simulink model "schema_controllo_attritoStatico_CompDist"  (Simulink 8.8)
settings: Solver=VariableStepAuto  StartTime=0.0  StopTime=Tf  FixedStep=T  MaxStep=T  RelTol=1e-3  EnableMultiTasking=on
values from neighbouring files (symbols this model uses):
  Kr = diag(kr)    [calcolaDisturbo.m]
undefined symbols (not defined in the file or in its folder): bmStim, calcolaDisturboStim, dqData, Ka, km, Kp, kt, kta, ktp, ktv, Kv, kv, qData, Ra, T, Ta
CloseFcn:
  | rtwprivate ssgencode ModelCloseRequest ContributiCoppieComau
settings Model: Creator=Alessandro  LastModifiedBy=joecr  ExtModeAutoUpdateStatusClock=off
settings DataIOCC: OutputOption=SpecifiedOutputTimes  OutputTimes=[Ti:T:Tf]
settings OptimizationCC: ExpressionDepthLimit=2147483647  InitFltsAndDblsToZero=on
settings DebuggingCC: AlgebraicLoopMsg=none  SaveWithParameterizedLinksMsg=none  SignalResolutionControl=TryResolveAllWithWarning  SolverPrmCheckMsg=warning  InheritedTsInSrcMsg=none  MultiTaskDSMMsg=warning  MultiTaskCondExecSysMsg=none  TasksWithSamePriorityMsg=none  AllowSymbolicDim=off
settings GRTTargetCC: TargetFcnLib=ansi_tfl_tmw.mat

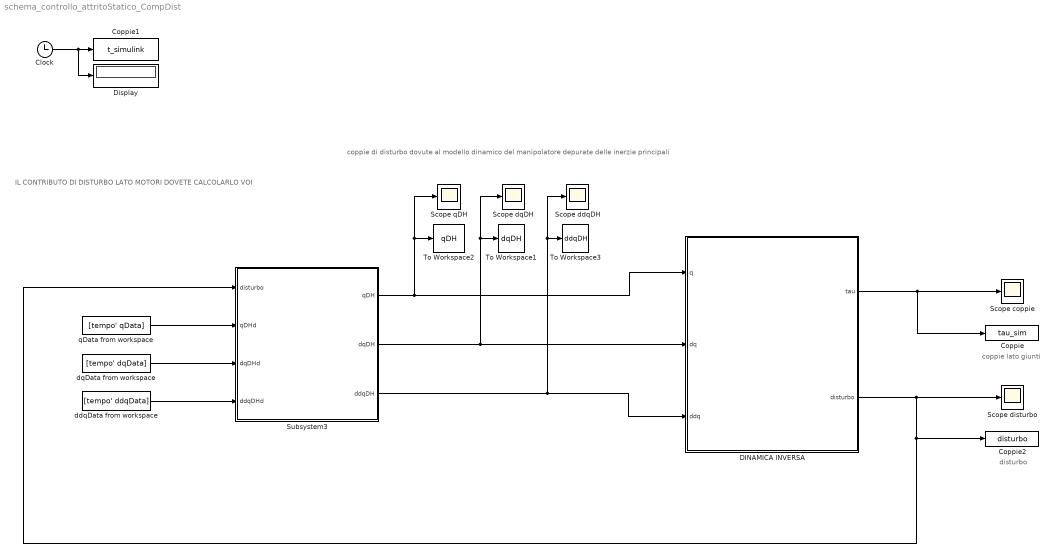
== system schema_controllo_attritoStatico_CompDist ==
  note: coppie di disturbo dovute al modello dinamico del manipolatore depurate delle inerzie principali
  note: coppie lato giunti
  note: IL CONTRIBUTO DI DISTURBO LATO MOTORI DOVETE CALCOLARLO VOI
  note: disturbo
  Clock : Clock
  Coppie : ToWorkspace  VariableName=tau_sim  SampleTime=-1
  Coppie1 : ToWorkspace  VariableName=t_simulink  SampleTime=-1
  Coppie2 : ToWorkspace  VariableName=disturbo  SampleTime=-1
  DINAMICA INVERSA : Subsystem
      mask Display:
      | disp('Contributi Coppie');
      | port_label('input', 1, 'qDH');
      | port_label('input', 2, 'dqDH');
      | port_label('input', 3, 'ddqDH');
      | port_label('output', 1, 'Coppie Complessive');
      | port_label('output', 2, 'Disturbo lato motori');
  Display : Display
  Scope coppie : Scope
  Scope ddqDH : Scope
  Scope disturbo : Scope
  Scope dqDH : Scope
  Scope qDH : Scope
  Subsystem3 : Subsystem
      mask Display:
      | disp('Controllo');
      | port_label('input', 1, 'disturbo');
      | port_label('input', 2, 'qDHd');
      | port_label('input', 3, 'dqDHd');
      | port_label('input', 4, 'ddqDHd');
      | port_label('output', 1, 'qDH');
      | port_label('output', 2, 'dqDH');
      | port_label('output', 3, 'ddqDH');
  To Workspace1 : ToWorkspace  VariableName=dqDH  SampleTime=-1
  To Workspace2 : ToWorkspace  VariableName=qDH  SampleTime=-1
  To Workspace3 : ToWorkspace  VariableName=ddqDH  SampleTime=-1
  ddqData from workspace : FromWorkspace  VariableName=[tempo' ddqData]  OutputAfterFinalValue=Holding final value
  dqData from workspace : FromWorkspace  VariableName=[tempo' dqData]  OutputAfterFinalValue=Holding final value
  qData from workspace : FromWorkspace  VariableName=[tempo' qData]  OutputAfterFinalValue=Holding final value
  wires:
  Clock/1 -> Coppie1/1, Display/1
  Subsystem3/2(dqDH) -> To Workspace1/1, Scope dqDH/1, DINAMICA INVERSA/2(dq)
  DINAMICA INVERSA/1(tau) -> Coppie/1, Scope coppie/1
  Subsystem3/1(qDH) -> DINAMICA INVERSA/1(q), To Workspace2/1, Scope qDH/1
  Subsystem3/3(ddqDH) -> DINAMICA INVERSA/3(ddq), To Workspace3/1, Scope ddqDH/1
  DINAMICA INVERSA/2(disturbo) -> Subsystem3/1(disturbo), Coppie2/1, Scope disturbo/1
  qData from workspace/1 -> Subsystem3/2(qDHd)
  dqData from workspace/1 -> Subsystem3/3(dqDHd)
  ddqData from workspace/1 -> Subsystem3/4(ddqDHd)

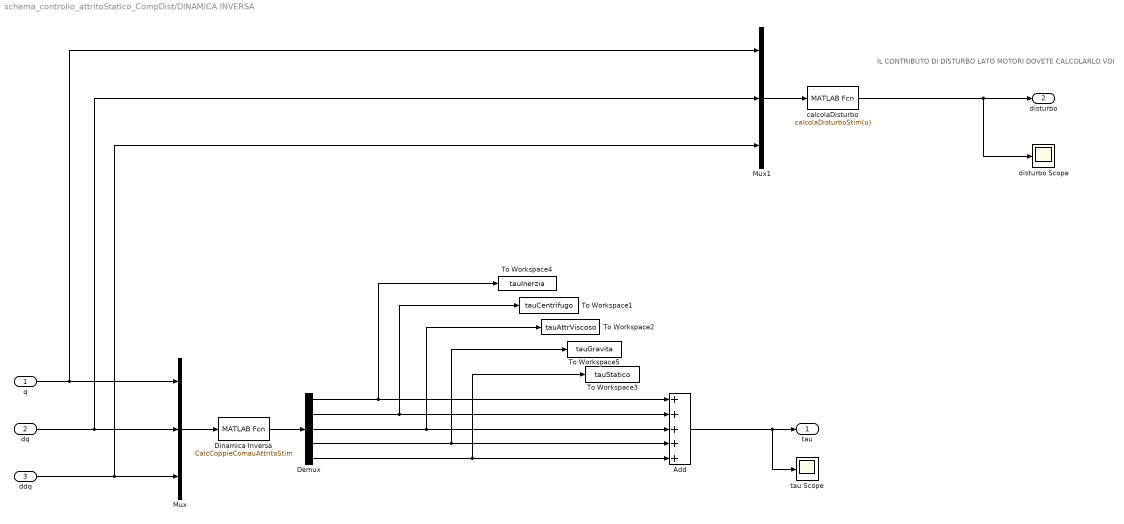
== system schema_controllo_attritoStatico_CompDist/DINAMICA INVERSA ==
  note: IL CONTRIBUTO DI DISTURBO LATO MOTORI DOVETE CALCOLARLO VOI
  q : Inport
  dq : Inport  Port=2
  ddq : Inport  Port=3
  Add : Sum  Inputs=+++++
  Demux : Demux  Outputs=5
  Dinamica Inversa : MATLABFcn  MATLABFcn=CalcCoppieComauAttritoStim  OutputDimensions=30
  Mux : Mux  Inputs=3
  Mux1 : Mux  Inputs=3
  To Workspace1 : ToWorkspace  VariableName=tauCentrifugo  SampleTime=-1
  To Workspace2 : ToWorkspace  VariableName=tauAttrViscoso  SampleTime=-1
  To Workspace3 : ToWorkspace  VariableName=tauStatico  SampleTime=-1
  To Workspace4 : ToWorkspace  VariableName=tauInerzia  SampleTime=-1
  To Workspace5 : ToWorkspace  VariableName=tauGravita  SampleTime=-1
  calcolaDisturbo : MATLABFcn  MATLABFcn=calcolaDisturboStim(u)  OutputDimensions=6
  disturbo Scope : Scope
  tau Scope : Scope
  tau : Outport
  disturbo : Outport  Port=2
  wires:
  Mux/1 -> Dinamica Inversa/1
  ddq/1 -> Mux1/3, Mux/3
  Dinamica Inversa/1 -> Demux/1
  Demux/1 -> To Workspace4/1, Add/1
  Demux/3 -> Add/3, To Workspace2/1
  Demux/4 -> Add/4, To Workspace5/1
  calcolaDisturbo/1 -> disturbo Scope/1, disturbo/1
  Mux1/1 -> calcolaDisturbo/1
  Demux/2 -> Add/2, To Workspace1/1
  Add/1 -> tau Scope/1, tau/1
  q/1 -> Mux1/1, Mux/1
  dq/1 -> Mux1/2, Mux/2
  Demux/5 -> To Workspace3/1, Add/5

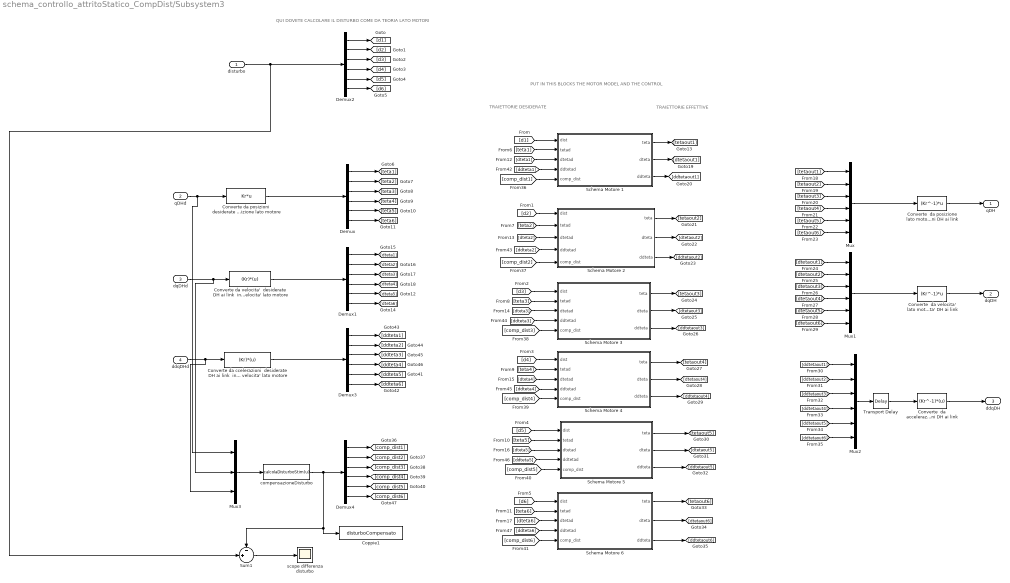
== system schema_controllo_attritoStatico_CompDist/Subsystem3 ==
  note: PUT IN THIS BLOCKS THE MOTOR MODEL AND THE CONTROL
  note: TRAIETTORIE DESIDERATE
  note: TRAIETTORIE EFFETTIVE
  note: QUI DOVETE CALCOLARE IL DISTURBO COME DA TEORIA LATO MOTORI
  disturbo : Inport
  qDHd : Inport  Port=2
  dqDHd : Inport  Port=3
  ddqDHd : Inport  Port=4
  Converte  da accelerazioni lato motore  ad accelerazioni DH ai link : MATLABFcn  MATLABFcn=(Kr^-1)*(u)
  "Converte  da posizione lato motore a  posizioni DH ai link " : MATLABFcn  MATLABFcn=(Kr^-1)*u
  "Converte  da velocita' lato motore  a velocita' DH ai link " : MATLABFcn  MATLABFcn=(Kr^-1)*u
  Converte da ccelerazioni  desiderate DH ai link  in velocita' lato motore : MATLABFcn  MATLABFcn=(Kr)*(u)
  "Converte da posizioni  desiderate DH ai link  in posizione lato motore " : MATLABFcn  MATLABFcn=Kr*u
  "Converte da velocita'  desiderate DH ai link  in velocita' lato motore " : MATLABFcn  MATLABFcn=(Kr)*(u)
  Coppie1 : ToWorkspace  VariableName=disturboCompensato  SampleTime=-1
  Demux{,1..4} (5 alike) : Demux  Outputs=6
  Mux : Mux  Inputs=6
  Mux1 : Mux  Inputs=6
  Mux2 : Mux  Inputs=6
  Mux3 : Mux  Inputs=3
  Schema Motore 1 : Subsystem  mask{i=1}
  Schema Motore 2 : Subsystem  mask{i=2}
  Schema Motore 3 : Subsystem  mask{i=3}
  Schema Motore 4 : Subsystem  mask{i=4}
  Schema Motore 5 : Subsystem  mask{i=5}
  Schema Motore 6 : Subsystem  mask{i=6}
  Sum1 : Sum  Inputs=-+|
  Transport Delay : TransportDelay  DelayTime=T
  compensazioneDisturbo : MATLABFcn  MATLABFcn=calcolaDisturboStim(u)
  scope differenza disturbo : Scope
  qDH : Outport
  dqDH : Outport  Port=2
  ddqDH : Outport  Port=3
  wires:
  qDHd/1 -> Mux3/1, "Converte da posizioni  desiderate DH ai link  in posizione lato motore "/1
  dqDHd/1 -> Mux3/2, "Converte da velocita'  desiderate DH ai link  in velocita' lato motore "/1
  "Converte  da velocita' lato motore  a velocita' DH ai link "/1 -> dqDH/1
  Converte  da accelerazioni lato motore  ad accelerazioni DH ai link/1 -> ddqDH/1
  "Converte da posizioni  desiderate DH ai link  in posizione lato motore "/1 -> Demux/1
  disturbo/1 -> Sum1/2, Demux2/1
  "Converte  da posizione lato motore a  posizioni DH ai link "/1 -> qDH/1
  Mux/1 -> "Converte  da posizione lato motore a  posizioni DH ai link "/1
  Demux2/1 -> [d1]
  Demux2/2 -> [d2]
  Demux2/3 -> [d3]
  Demux2/4 -> [d4]
  Demux2/5 -> [d5]
  Demux2/6 -> [d6]
  [d3] -> Schema Motore 3/1(dist)
  [d4] -> Schema Motore 4/1(dist)
  [d5] -> Schema Motore 5/1(dist)
  [d6] -> Schema Motore 6/1(dist)
  Demux/1 -> [teta1]
  Demux/2 -> [teta2]
  Demux/3 -> [teta3]
  Demux/4 -> [teta4]
  Demux/5 -> [teta5]
  Demux/6 -> [teta6]
  [teta2] -> Schema Motore 2/2(tetad)
  [teta3] -> Schema Motore 3/2(tetad)
  [teta4] -> Schema Motore 4/2(tetad)
  [teta5] -> Schema Motore 5/2(tetad)
  [teta6] -> Schema Motore 6/2(tetad)
  "Converte da velocita'  desiderate DH ai link  in velocita' lato motore "/1 -> Demux1/1
  Demux1/1 -> [dteta1]
  Demux1/2 -> [dteta2]
  Demux1/3 -> [dteta3]
  Demux1/4 -> [dteta4]
  Demux1/5 -> [dteta5]
  Demux1/6 -> [dteta6]
  [dteta2] -> Schema Motore 2/3(dtetad)
  [tetaout1] -> Mux/1
  [tetaout2] -> Mux/2
  [tetaout3] -> Mux/3
  [tetaout4] -> Mux/4
  [tetaout5] -> Mux/5
  [tetaout6] -> Mux/6
  Mux1/1 -> "Converte  da velocita' lato motore  a velocita' DH ai link "/1
  [dtetaout1] -> Mux1/1
  [dtetaout2] -> Mux1/2
  [dtetaout3] -> Mux1/3
  [dtetaout4] -> Mux1/4
  [dtetaout5] -> Mux1/5
  [dtetaout6] -> Mux1/6
  Mux2/1 -> Transport Delay/1
  [ddtetaout1] -> Mux2/1
  [ddtetaout2] -> Mux2/2
  [ddtetaout3] -> Mux2/3
  [ddtetaout4] -> Mux2/4
  [ddtetaout5] -> Mux2/5
  [ddtetaout6] -> Mux2/6
  Schema Motore 2/1(teta) -> [tetaout2]
  Schema Motore 2/2(dteta) -> [dtetaout2]
  Transport Delay/1 -> Converte  da accelerazioni lato motore  ad accelerazioni DH ai link/1
  [teta1] -> Schema Motore 1/2(tetad)
  [dteta1] -> Schema Motore 1/3(dtetad)
  Schema Motore 1/1(teta) -> [tetaout1]
  Schema Motore 1/2(dteta) -> [dtetaout1]
  Schema Motore 1/3(ddteta) -> [ddtetaout1]
  [d1] -> Schema Motore 1/1(dist)
  ddqDHd/1 -> Mux3/3, Converte da ccelerazioni  desiderate DH ai link  in velocita' lato motore/1
  Demux3/1 -> [ddteta1]
  Demux3/2 -> [ddteta2]
  Demux3/3 -> [ddteta3]
  Demux3/4 -> [ddteta4]
  Demux3/5 -> [ddteta5]
  Demux3/6 -> [ddteta6]
  Converte da ccelerazioni  desiderate DH ai link  in velocita' lato motore/1 -> Demux3/1
  [ddteta1] -> Schema Motore 1/4(ddtetad)
  Schema Motore 3/1(teta) -> [tetaout3]
  Schema Motore 3/2(dteta) -> [dtetaout3]
  Schema Motore 3/3(ddteta) -> [ddtetaout3]
  Schema Motore 4/1(teta) -> [tetaout4]
  Schema Motore 4/2(dteta) -> [dtetaout4]
  Schema Motore 4/3(ddteta) -> [ddtetaout4]
  Schema Motore 5/1(teta) -> [tetaout5]
  Schema Motore 5/2(dteta) -> [dtetaout5]
  Schema Motore 5/3(ddteta) -> [ddtetaout5]
  Schema Motore 6/1(teta) -> [tetaout6]
  Schema Motore 6/2(dteta) -> [dtetaout6]
  Schema Motore 6/3(ddteta) -> [ddtetaout6]
  [ddteta2] -> Schema Motore 2/4(ddtetad)
  [dteta4] -> Schema Motore 4/3(dtetad)
  [ddteta4] -> Schema Motore 4/4(ddtetad)
  [ddteta3] -> Schema Motore 3/4(ddtetad)
  [dteta3] -> Schema Motore 3/3(dtetad)
  [d2] -> Schema Motore 2/1(dist)
  Schema Motore 2/3(ddteta) -> [ddtetaout2]
  [dteta5] -> Schema Motore 5/3(dtetad)
  [ddteta5] -> Schema Motore 5/4(ddtetad)
  [dteta6] -> Schema Motore 6/3(dtetad)
  [ddteta6] -> Schema Motore 6/4(ddtetad)
  [comp_dist1] -> Schema Motore 1/5(comp_dist)
  Demux4/1 -> [comp_dist1]
  Demux4/2 -> [comp_dist2]
  Demux4/3 -> [comp_dist3]
  Demux4/4 -> [comp_dist4]
  Demux4/5 -> [comp_dist5]
  Demux4/6 -> [comp_dist6]
  Mux3/1 -> compensazioneDisturbo/1
  [comp_dist2] -> Schema Motore 2/5(comp_dist)
  [comp_dist6] -> Schema Motore 6/5(comp_dist)
  [comp_dist5] -> Schema Motore 5/5(comp_dist)
  [comp_dist4] -> Schema Motore 4/5(comp_dist)
  [comp_dist3] -> Schema Motore 3/5(comp_dist)
  compensazioneDisturbo/1 -> Sum1/1, Coppie1/1, Demux4/1
  Sum1/1 -> scope differenza disturbo/1

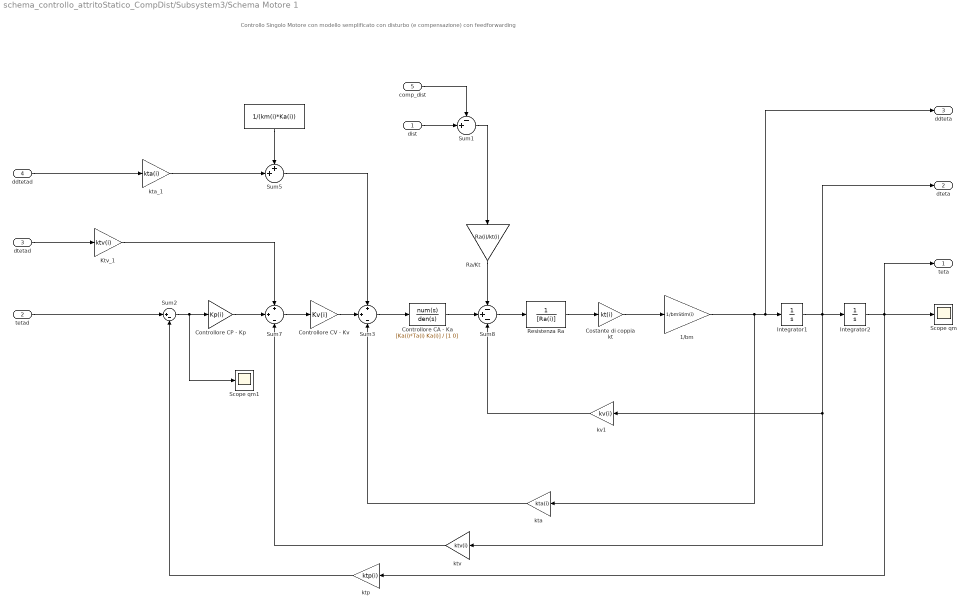
== system schema_controllo_attritoStatico_CompDist/Subsystem3/Schema Motore 1 ==
  note: Controllo Singolo Motore con modello semplificato con disturbo (e compensazione) con feedforwarding
  dist : Inport  PortDimensions=1
  tetad : Inport  Port=2  PortDimensions=1
  dtetad : Inport  Port=3  PortDimensions=1
  ddtetad : Inport  Port=4  PortDimensions=1
  comp_dist : Inport  Port=5  PortDimensions=1
  " " : Constant  Value=1/(km(i)*Ka(i))
  " Controllore CV - Kv" : Gain  Gain=Kv(i)
  1/bm : Gain  Gain=1/bmStim(i)
  Controllore CA - Ka : TransferFcn  Numerator=[Ka(i)*Ta(i) Ka(i)]  Denominator=[1 0]
  Controllore CP - Kp : Gain  Gain=Kp(i)
  Costante di coppia kt : Gain  Gain=kt(i)
  Integrator1 : Integrator  InitialCondition=Kr(i,i)*dqData(1,i)
  "Integrator2 " : Integrator  InitialCondition=Kr(i,i)*qData(1,i)
  Ktv_1 : Gain  Gain=ktv(i)
  Ra/Kt : Gain  Gain=Ra(i)/kt(i)
  "Resistenza Ra " : TransferFcn  Denominator=[Ra(i)]
  Scope qm : Scope
  Scope qm1 : Scope
  Sum1 : Sum  Inputs=-+|
  Sum2 : Sum  Inputs=|+-
  Sum3 : Sum  Inputs=+|+|-
  Sum5 : Sum  Inputs=++|
  Sum7 : Sum  Inputs=+|+|-
  Sum8 : Sum  Inputs=-+-
  kta : Gain  Gain=kta(i)
  kta_1 : Gain  Gain=kta(i)
  ktp : Gain  Gain=ktp(i)
  ktv : Gain  Gain=ktv(i)
  kv1 : Gain  Gain=kv(i)
  teta : Outport  PortDimensions=1
  dteta : Outport  Port=2  PortDimensions=1
  ddteta : Outport  Port=3  PortDimensions=1
  wires:
  Sum7/1 -> " Controllore CV - Kv"/1
  Sum3/1 -> Controllore CA - Ka/1
  ktp/1 -> Sum2/2
  tetad/1 -> Sum2/1
  Sum8/1 -> "Resistenza Ra "/1
  kv1/1 -> Sum8/3
  Integrator1/1 -> dteta/1, ktv/1, kv1/1, "Integrator2 "/1
  "Resistenza Ra "/1 -> Costante di coppia kt/1
  Costante di coppia kt/1 -> 1/bm/1
  Controllore CP - Kp/1 -> Sum7/2
  Ktv_1/1 -> Sum7/1
  ktv/1 -> Sum7/3
  " Controllore CV - Kv"/1 -> Sum3/2
  kta_1/1 -> Sum5/2
  " "/1 -> Sum5/1
  Sum5/1 -> Sum3/1
  ddtetad/1 -> kta_1/1
  dtetad/1 -> Ktv_1/1
  "Integrator2 "/1 -> ktp/1, teta/1, Scope qm/1
  kta/1 -> Sum3/3
  1/bm/1 -> kta/1, ddteta/1, Integrator1/1
  Ra/Kt/1 -> Sum8/1
  Controllore CA - Ka/1 -> Sum8/2
  comp_dist/1 -> Sum1/1
  Sum2/1 -> Scope qm1/1, Controllore CP - Kp/1
  dist/1 -> Sum1/2
  Sum1/1 -> Ra/Kt/1

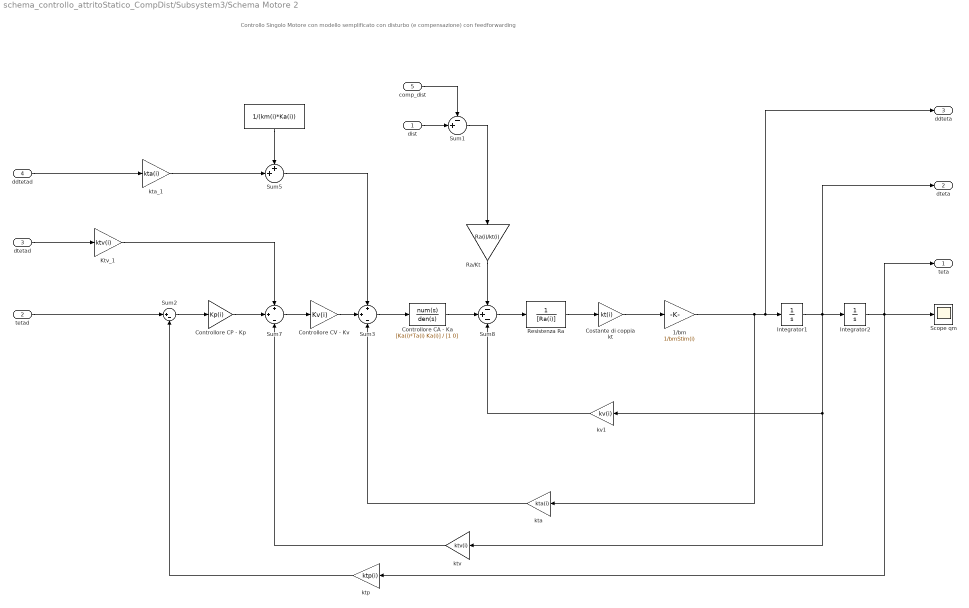
== system schema_controllo_attritoStatico_CompDist/Subsystem3/Schema Motore 2 ==
  note: Controllo Singolo Motore con modello semplificato con disturbo (e compensazione) con feedforwarding
  dist : Inport  PortDimensions=1
  tetad : Inport  Port=2  PortDimensions=1
  dtetad : Inport  Port=3  PortDimensions=1
  ddtetad : Inport  Port=4  PortDimensions=1
  comp_dist : Inport  Port=5  PortDimensions=1
  " " : Constant  Value=1/(km(i)*Ka(i))
  " Controllore CV - Kv" : Gain  Gain=Kv(i)
  1/bm : Gain  Gain=1/bmStim(i)
  Controllore CA - Ka : TransferFcn  Numerator=[Ka(i)*Ta(i) Ka(i)]  Denominator=[1 0]
  Controllore CP - Kp : Gain  Gain=Kp(i)
  Costante di coppia kt : Gain  Gain=kt(i)
  Integrator1 : Integrator  InitialCondition=Kr(i,i)*dqData(1,i)
  "Integrator2 " : Integrator  InitialCondition=Kr(i,i)*qData(1,i)
  Ktv_1 : Gain  Gain=ktv(i)
  Ra/Kt : Gain  Gain=Ra(i)/kt(i)
  "Resistenza Ra " : TransferFcn  Denominator=[Ra(i)]
  Scope qm : Scope
  Sum1 : Sum  Inputs=-+|
  Sum2 : Sum  Inputs=|+-
  Sum3 : Sum  Inputs=+|+|-
  Sum5 : Sum  Inputs=++|
  Sum7 : Sum  Inputs=+|+|-
  Sum8 : Sum  Inputs=-+-
  kta : Gain  Gain=kta(i)
  kta_1 : Gain  Gain=kta(i)
  ktp : Gain  Gain=ktp(i)
  ktv : Gain  Gain=ktv(i)
  kv1 : Gain  Gain=kv(i)
  teta : Outport  PortDimensions=1
  dteta : Outport  Port=2  PortDimensions=1
  ddteta : Outport  Port=3  PortDimensions=1
  wires:
  Sum7/1 -> " Controllore CV - Kv"/1
  Sum3/1 -> Controllore CA - Ka/1
  ktp/1 -> Sum2/2
  tetad/1 -> Sum2/1
  Sum8/1 -> "Resistenza Ra "/1
  kv1/1 -> Sum8/3
  Integrator1/1 -> dteta/1, ktv/1, kv1/1, "Integrator2 "/1
  "Resistenza Ra "/1 -> Costante di coppia kt/1
  Costante di coppia kt/1 -> 1/bm/1
  Controllore CP - Kp/1 -> Sum7/2
  Ktv_1/1 -> Sum7/1
  ktv/1 -> Sum7/3
  " Controllore CV - Kv"/1 -> Sum3/2
  kta_1/1 -> Sum5/2
  " "/1 -> Sum5/1
  Sum5/1 -> Sum3/1
  ddtetad/1 -> kta_1/1
  dtetad/1 -> Ktv_1/1
  "Integrator2 "/1 -> ktp/1, teta/1, Scope qm/1
  kta/1 -> Sum3/3
  Sum2/1 -> Controllore CP - Kp/1
  1/bm/1 -> ddteta/1, Integrator1/1, kta/1
  Ra/Kt/1 -> Sum8/1
  Controllore CA - Ka/1 -> Sum8/2
  dist/1 -> Sum1/2
  comp_dist/1 -> Sum1/1
  Sum1/1 -> Ra/Kt/1

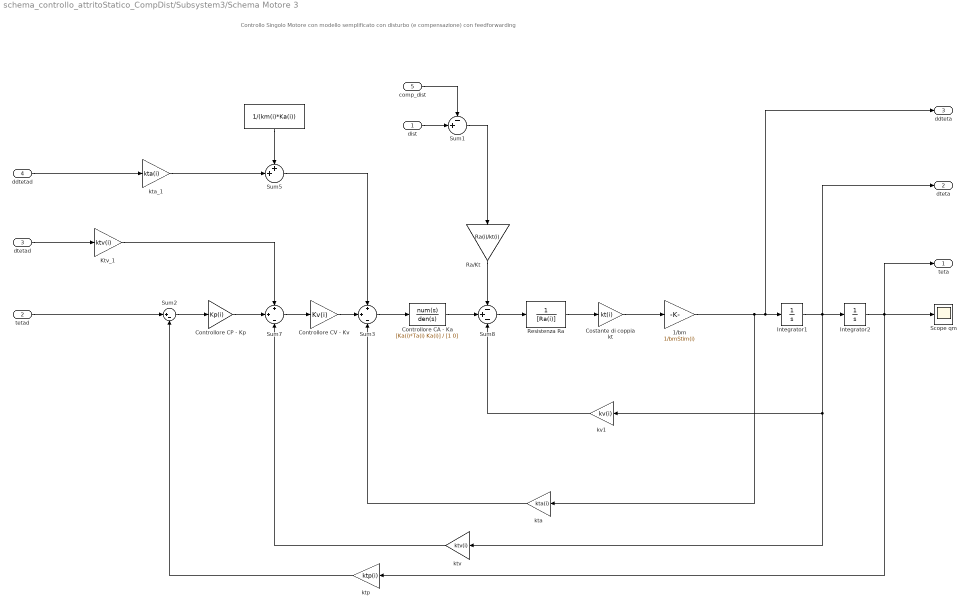
== system schema_controllo_attritoStatico_CompDist/Subsystem3/Schema Motore 3 ==
  note: Controllo Singolo Motore con modello semplificato con disturbo (e compensazione) con feedforwarding
  dist : Inport  PortDimensions=1
  tetad : Inport  Port=2  PortDimensions=1
  dtetad : Inport  Port=3  PortDimensions=1
  ddtetad : Inport  Port=4  PortDimensions=1
  comp_dist : Inport  Port=5  PortDimensions=1
  " " : Constant  Value=1/(km(i)*Ka(i))
  " Controllore CV - Kv" : Gain  Gain=Kv(i)
  1/bm : Gain  Gain=1/bmStim(i)
  Controllore CA - Ka : TransferFcn  Numerator=[Ka(i)*Ta(i) Ka(i)]  Denominator=[1 0]
  Controllore CP - Kp : Gain  Gain=Kp(i)
  Costante di coppia kt : Gain  Gain=kt(i)
  Integrator1 : Integrator  InitialCondition=Kr(i,i)*dqData(1,i)
  "Integrator2 " : Integrator  InitialCondition=Kr(i,i)*qData(1,i)
  Ktv_1 : Gain  Gain=ktv(i)
  Ra/Kt : Gain  Gain=Ra(i)/kt(i)
  "Resistenza Ra " : TransferFcn  Denominator=[Ra(i)]
  Scope qm : Scope
  Sum1 : Sum  Inputs=-+|
  Sum2 : Sum  Inputs=|+-
  Sum3 : Sum  Inputs=+|+|-
  Sum5 : Sum  Inputs=++|
  Sum7 : Sum  Inputs=+|+|-
  Sum8 : Sum  Inputs=-+-
  kta : Gain  Gain=kta(i)
  kta_1 : Gain  Gain=kta(i)
  ktp : Gain  Gain=ktp(i)
  ktv : Gain  Gain=ktv(i)
  kv1 : Gain  Gain=kv(i)
  teta : Outport  PortDimensions=1
  dteta : Outport  Port=2  PortDimensions=1
  ddteta : Outport  Port=3  PortDimensions=1
  wires:
  Sum7/1 -> " Controllore CV - Kv"/1
  Sum3/1 -> Controllore CA - Ka/1
  ktp/1 -> Sum2/2
  tetad/1 -> Sum2/1
  Sum8/1 -> "Resistenza Ra "/1
  kv1/1 -> Sum8/3
  Integrator1/1 -> dteta/1, ktv/1, kv1/1, "Integrator2 "/1
  "Resistenza Ra "/1 -> Costante di coppia kt/1
  Costante di coppia kt/1 -> 1/bm/1
  Controllore CP - Kp/1 -> Sum7/2
  Ktv_1/1 -> Sum7/1
  ktv/1 -> Sum7/3
  " Controllore CV - Kv"/1 -> Sum3/2
  kta_1/1 -> Sum5/2
  " "/1 -> Sum5/1
  Sum5/1 -> Sum3/1
  ddtetad/1 -> kta_1/1
  dtetad/1 -> Ktv_1/1
  "Integrator2 "/1 -> ktp/1, teta/1, Scope qm/1
  kta/1 -> Sum3/3
  Sum2/1 -> Controllore CP - Kp/1
  1/bm/1 -> ddteta/1, Integrator1/1, kta/1
  Ra/Kt/1 -> Sum8/1
  Controllore CA - Ka/1 -> Sum8/2
  dist/1 -> Sum1/2
  comp_dist/1 -> Sum1/1
  Sum1/1 -> Ra/Kt/1

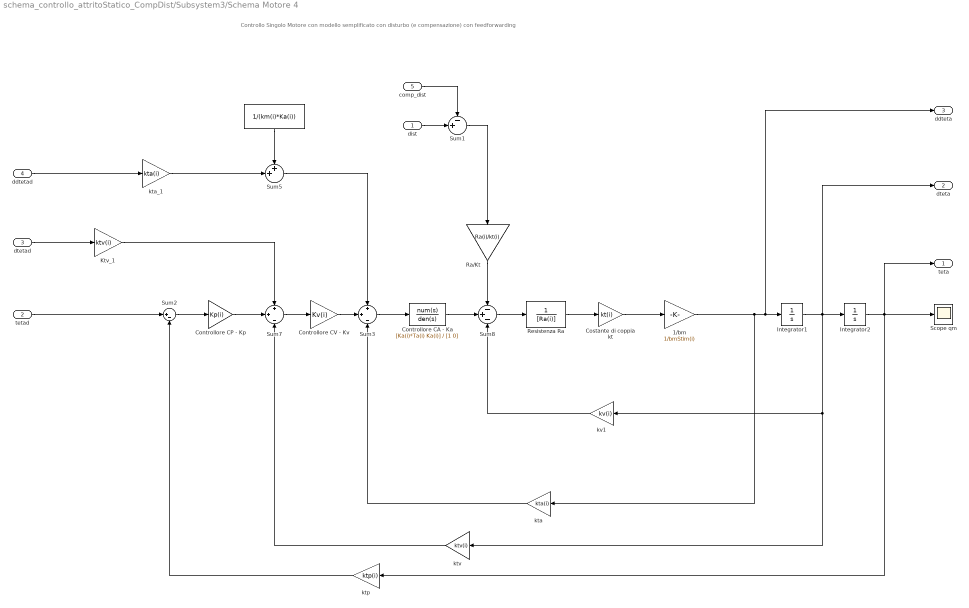
== system schema_controllo_attritoStatico_CompDist/Subsystem3/Schema Motore 4 ==
  note: Controllo Singolo Motore con modello semplificato con disturbo (e compensazione) con feedforwarding
  dist : Inport  PortDimensions=1
  tetad : Inport  Port=2  PortDimensions=1
  dtetad : Inport  Port=3  PortDimensions=1
  ddtetad : Inport  Port=4  PortDimensions=1
  comp_dist : Inport  Port=5  PortDimensions=1
  " " : Constant  Value=1/(km(i)*Ka(i))
  " Controllore CV - Kv" : Gain  Gain=Kv(i)
  1/bm : Gain  Gain=1/bmStim(i)
  Controllore CA - Ka : TransferFcn  Numerator=[Ka(i)*Ta(i) Ka(i)]  Denominator=[1 0]
  Controllore CP - Kp : Gain  Gain=Kp(i)
  Costante di coppia kt : Gain  Gain=kt(i)
  Integrator1 : Integrator  InitialCondition=Kr(i,i)*dqData(1,i)
  "Integrator2 " : Integrator  InitialCondition=Kr(i,i)*qData(1,i)
  Ktv_1 : Gain  Gain=ktv(i)
  Ra/Kt : Gain  Gain=Ra(i)/kt(i)
  "Resistenza Ra " : TransferFcn  Denominator=[Ra(i)]
  Scope qm : Scope
  Sum1 : Sum  Inputs=-+|
  Sum2 : Sum  Inputs=|+-
  Sum3 : Sum  Inputs=+|+|-
  Sum5 : Sum  Inputs=++|
  Sum7 : Sum  Inputs=+|+|-
  Sum8 : Sum  Inputs=-+-
  kta : Gain  Gain=kta(i)
  kta_1 : Gain  Gain=kta(i)
  ktp : Gain  Gain=ktp(i)
  ktv : Gain  Gain=ktv(i)
  kv1 : Gain  Gain=kv(i)
  teta : Outport  PortDimensions=1
  dteta : Outport  Port=2  PortDimensions=1
  ddteta : Outport  Port=3  PortDimensions=1
  wires:
  Sum7/1 -> " Controllore CV - Kv"/1
  Sum3/1 -> Controllore CA - Ka/1
  ktp/1 -> Sum2/2
  tetad/1 -> Sum2/1
  Sum8/1 -> "Resistenza Ra "/1
  kv1/1 -> Sum8/3
  Integrator1/1 -> dteta/1, ktv/1, kv1/1, "Integrator2 "/1
  "Resistenza Ra "/1 -> Costante di coppia kt/1
  Costante di coppia kt/1 -> 1/bm/1
  Controllore CP - Kp/1 -> Sum7/2
  Ktv_1/1 -> Sum7/1
  ktv/1 -> Sum7/3
  " Controllore CV - Kv"/1 -> Sum3/2
  kta_1/1 -> Sum5/2
  " "/1 -> Sum5/1
  Sum5/1 -> Sum3/1
  ddtetad/1 -> kta_1/1
  dtetad/1 -> Ktv_1/1
  "Integrator2 "/1 -> ktp/1, teta/1, Scope qm/1
  kta/1 -> Sum3/3
  Sum2/1 -> Controllore CP - Kp/1
  1/bm/1 -> ddteta/1, Integrator1/1, kta/1
  Ra/Kt/1 -> Sum8/1
  Controllore CA - Ka/1 -> Sum8/2
  dist/1 -> Sum1/2
  comp_dist/1 -> Sum1/1
  Sum1/1 -> Ra/Kt/1

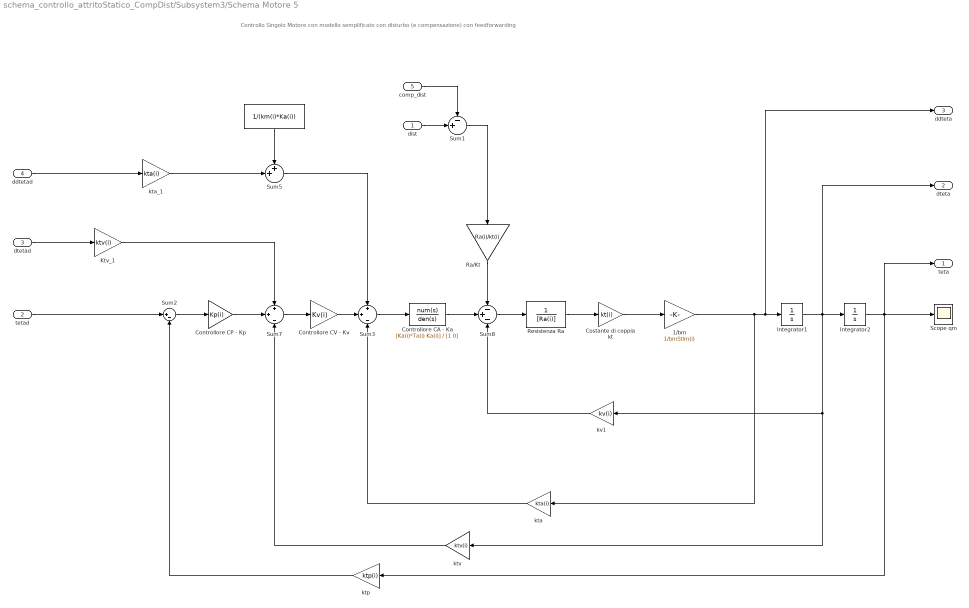
== system schema_controllo_attritoStatico_CompDist/Subsystem3/Schema Motore 5 ==
  note: Controllo Singolo Motore con modello semplificato con disturbo (e compensazione) con feedforwarding
  dist : Inport  PortDimensions=1
  tetad : Inport  Port=2  PortDimensions=1
  dtetad : Inport  Port=3  PortDimensions=1
  ddtetad : Inport  Port=4  PortDimensions=1
  comp_dist : Inport  Port=5  PortDimensions=1
  " " : Constant  Value=1/(km(i)*Ka(i))
  " Controllore CV - Kv" : Gain  Gain=Kv(i)
  1/bm : Gain  Gain=1/bmStim(i)
  Controllore CA - Ka : TransferFcn  Numerator=[Ka(i)*Ta(i) Ka(i)]  Denominator=[1 0]
  Controllore CP - Kp : Gain  Gain=Kp(i)
  Costante di coppia kt : Gain  Gain=kt(i)
  Integrator1 : Integrator  InitialCondition=Kr(i,i)*dqData(1,i)
  "Integrator2 " : Integrator  InitialCondition=Kr(i,i)*qData(1,i)
  Ktv_1 : Gain  Gain=ktv(i)
  Ra/Kt : Gain  Gain=Ra(i)/kt(i)
  "Resistenza Ra " : TransferFcn  Denominator=[Ra(i)]
  Scope qm : Scope
  Sum1 : Sum  Inputs=-+|
  Sum2 : Sum  Inputs=|+-
  Sum3 : Sum  Inputs=+|+|-
  Sum5 : Sum  Inputs=++|
  Sum7 : Sum  Inputs=+|+|-
  Sum8 : Sum  Inputs=-+-
  kta : Gain  Gain=kta(i)
  kta_1 : Gain  Gain=kta(i)
  ktp : Gain  Gain=ktp(i)
  ktv : Gain  Gain=ktv(i)
  kv1 : Gain  Gain=kv(i)
  teta : Outport  PortDimensions=1
  dteta : Outport  Port=2  PortDimensions=1
  ddteta : Outport  Port=3  PortDimensions=1
  wires:
  Sum7/1 -> " Controllore CV - Kv"/1
  Sum3/1 -> Controllore CA - Ka/1
  ktp/1 -> Sum2/2
  tetad/1 -> Sum2/1
  Sum8/1 -> "Resistenza Ra "/1
  kv1/1 -> Sum8/3
  Integrator1/1 -> dteta/1, ktv/1, kv1/1, "Integrator2 "/1
  "Resistenza Ra "/1 -> Costante di coppia kt/1
  Costante di coppia kt/1 -> 1/bm/1
  Controllore CP - Kp/1 -> Sum7/2
  Ktv_1/1 -> Sum7/1
  ktv/1 -> Sum7/3
  " Controllore CV - Kv"/1 -> Sum3/2
  kta_1/1 -> Sum5/2
  " "/1 -> Sum5/1
  Sum5/1 -> Sum3/1
  ddtetad/1 -> kta_1/1
  dtetad/1 -> Ktv_1/1
  "Integrator2 "/1 -> ktp/1, teta/1, Scope qm/1
  kta/1 -> Sum3/3
  Sum2/1 -> Controllore CP - Kp/1
  1/bm/1 -> ddteta/1, Integrator1/1, kta/1
  Ra/Kt/1 -> Sum8/1
  Controllore CA - Ka/1 -> Sum8/2
  dist/1 -> Sum1/2
  comp_dist/1 -> Sum1/1
  Sum1/1 -> Ra/Kt/1

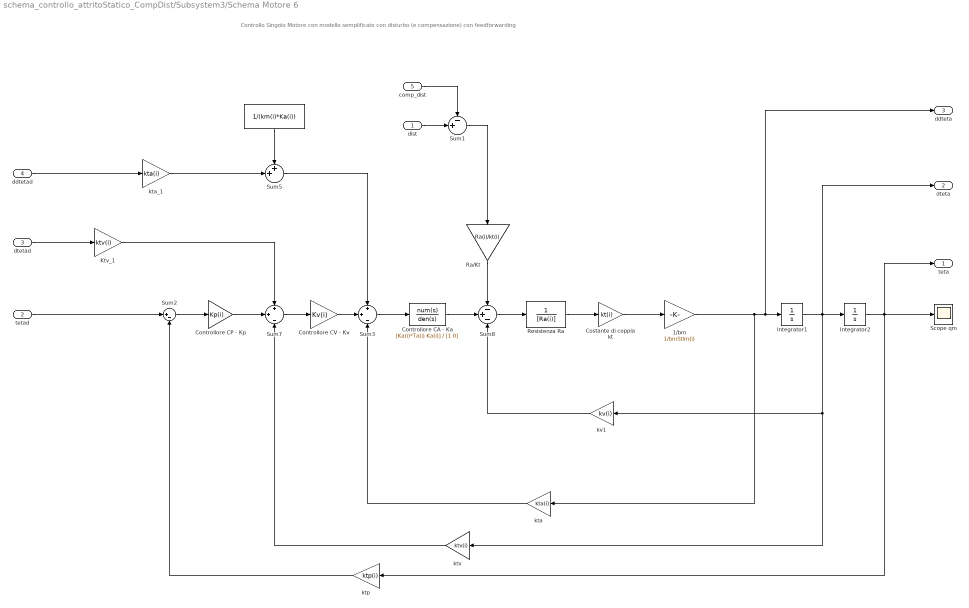
== system schema_controllo_attritoStatico_CompDist/Subsystem3/Schema Motore 6 ==
  note: Controllo Singolo Motore con modello semplificato con disturbo (e compensazione) con feedforwarding
  dist : Inport  PortDimensions=1
  tetad : Inport  Port=2  PortDimensions=1
  dtetad : Inport  Port=3  PortDimensions=1
  ddtetad : Inport  Port=4  PortDimensions=1
  comp_dist : Inport  Port=5  PortDimensions=1
  " " : Constant  Value=1/(km(i)*Ka(i))
  " Controllore CV - Kv" : Gain  Gain=Kv(i)
  1/bm : Gain  Gain=1/bmStim(i)
  Controllore CA - Ka : TransferFcn  Numerator=[Ka(i)*Ta(i) Ka(i)]  Denominator=[1 0]
  Controllore CP - Kp : Gain  Gain=Kp(i)
  Costante di coppia kt : Gain  Gain=kt(i)
  Integrator1 : Integrator  InitialCondition=Kr(i,i)*dqData(1,i)
  "Integrator2 " : Integrator  InitialCondition=Kr(i,i)*qData(1,i)
  Ktv_1 : Gain  Gain=ktv(i)
  Ra/Kt : Gain  Gain=Ra(i)/kt(i)
  "Resistenza Ra " : TransferFcn  Denominator=[Ra(i)]
  Scope qm : Scope
  Sum1 : Sum  Inputs=-+|
  Sum2 : Sum  Inputs=|+-
  Sum3 : Sum  Inputs=+|+|-
  Sum5 : Sum  Inputs=++|
  Sum7 : Sum  Inputs=+|+|-
  Sum8 : Sum  Inputs=-+-
  kta : Gain  Gain=kta(i)
  kta_1 : Gain  Gain=kta(i)
  ktp : Gain  Gain=ktp(i)
  ktv : Gain  Gain=ktv(i)
  kv1 : Gain  Gain=kv(i)
  teta : Outport  PortDimensions=1
  dteta : Outport  Port=2  PortDimensions=1
  ddteta : Outport  Port=3  PortDimensions=1
  wires:
  Sum7/1 -> " Controllore CV - Kv"/1
  Sum3/1 -> Controllore CA - Ka/1
  ktp/1 -> Sum2/2
  tetad/1 -> Sum2/1
  Sum8/1 -> "Resistenza Ra "/1
  kv1/1 -> Sum8/3
  Integrator1/1 -> dteta/1, ktv/1, kv1/1, "Integrator2 "/1
  "Resistenza Ra "/1 -> Costante di coppia kt/1
  Costante di coppia kt/1 -> 1/bm/1
  Controllore CP - Kp/1 -> Sum7/2
  Ktv_1/1 -> Sum7/1
  ktv/1 -> Sum7/3
  " Controllore CV - Kv"/1 -> Sum3/2
  kta_1/1 -> Sum5/2
  " "/1 -> Sum5/1
  Sum5/1 -> Sum3/1
  ddtetad/1 -> kta_1/1
  dtetad/1 -> Ktv_1/1
  "Integrator2 "/1 -> ktp/1, teta/1, Scope qm/1
  kta/1 -> Sum3/3
  Sum2/1 -> Controllore CP - Kp/1
  1/bm/1 -> ddteta/1, Integrator1/1, kta/1
  Ra/Kt/1 -> Sum8/1
  Controllore CA - Ka/1 -> Sum8/2
  dist/1 -> Sum1/2
  comp_dist/1 -> Sum1/1
  Sum1/1 -> Ra/Kt/1
